simulink model "Pendulum_model_linearization_torque"  (R2016a)
settings: Solver=ode45  StartTime=0.0  StopTime=10  RelTol=1e-3
model workspace: external: MATLAB File C:\Users\Dick\Documents\GitHub\control-system-lab\dick\Matlab\Pendulum simulation\params.m (data not in the file)
values from neighbouring files (symbols this model uses):
  k_m = 50    [linearization_by_hand.m]    (also in params.m = 41.0587; symbolic_derivation.m)
  tau_e = 0.03    [linearization_by_hand.m]    (also in params.m = 0.0312; symbolic_derivation.m)
settings Model: Creator=Nathan  LastModifiedBy=Dick
settings DataIOCC: InitialState=states  LimitDataPoints=on  LoadInitialState=on  SaveFormat=Array
settings DebuggingCC: AllowSymbolicDim=off
settings HardwareCC: ProdBitPerPointer=32  ProdLargestAtomicFloat=None  ProdIntDivRoundTo=Undefined  ProdEndianess=Unspecified  ProdWordSize=32  ProdHWDeviceType=32-bit Generic
settings ModelReferenceCC: PropagateSignalLabelsOutOfModel=off
settings ConfigComp: CovModelRefEnable=Off

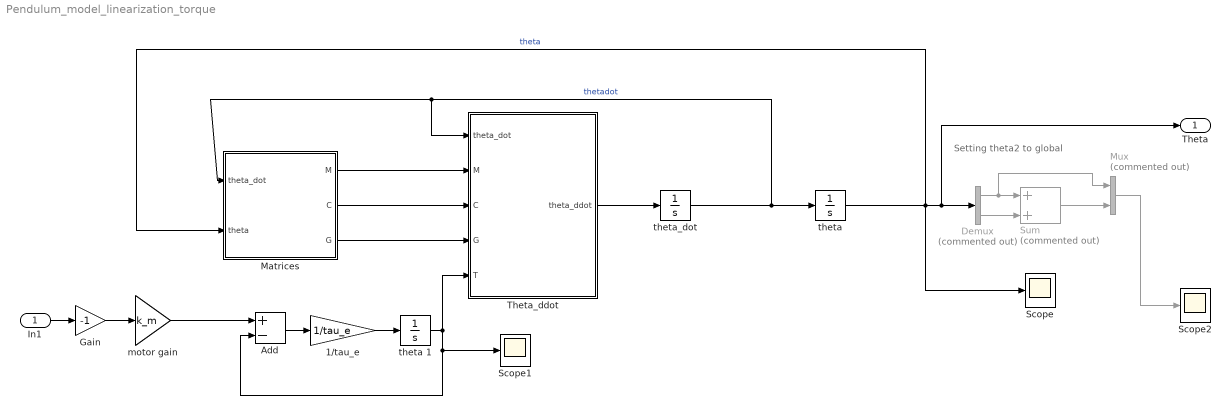
== system Pendulum_model_linearization_torque ==
  note: Setting theta2 to global
  In1 : Inport
  "1/tau_e " : Gain  Gain=1/tau_e
  Add : Sum  Inputs=+-
  Demux : Demux  Commented=on  Outputs=2
  Gain : Gain  Gain=-1
  Matrices : MATLAB Function  TreatAsAtomicUnit=on
  Mux : Mux  Commented=on  Inputs=2
  Scope : Scope
  Scope1 : Scope
  Scope2 : Scope
  Sum : Sum  Commented=on  Inputs=+|+
  "Theta_ddot " : MATLAB Function  TreatAsAtomicUnit=on
  "motor gain " : Gain  Gain=k_m
  "theta " : Integrator
  theta 1 : Integrator  ContinuousStateAttributes='torque'
  "theta_dot " : Integrator
  Theta : Outport
  wires:
  "theta "/1 -> Theta/1, Demux/1, Scope/1, Matrices/2(theta)  "theta"
  "theta_dot "/1 -> "theta "/1, "Theta_ddot "/1(theta_dot), Matrices/1(theta_dot)  "thetadot"
  "Theta_ddot "/1(theta_ddot) -> "theta_dot "/1
  Matrices/3(G) -> "Theta_ddot "/4(G)
  Matrices/2(C) -> "Theta_ddot "/3(C)
  Matrices/1(M) -> "Theta_ddot "/2(M)
  Demux/1 -> Mux/1, Sum/1
  Demux/2 -> Sum/2
  Sum/1 -> Mux/2
  Mux/1 -> Scope2/1
  In1/1 -> Gain/1
  theta 1/1 -> Scope1/1, Add/2, "Theta_ddot "/5(T)
  "1/tau_e "/1 -> theta 1/1
  Add/1 -> "1/tau_e "/1
  "motor gain "/1 -> Add/1
  Gain/1 -> "motor gain "/1

== matlab function Pendulum_model_linearization_torque/Theta_ddot  ==
  data: theta_dot input; M input; C input; G input; theta_ddot output; T input
function theta_ddot = fcn(theta_dot,M,C,G,T)
theta_ddot = [0;0];

theta_ddot = M\[T;0] - M\C*theta_dot - M\G;

== matlab function Pendulum_model_linearization_torque/Matrices ==
  data: theta_dot input; theta input; M output; C output; G output
function [M, C, G] = fcn(theta_dot, theta)

M = zeros(2);
C = zeros(2);
G = [0;0];

% %% Old parameters
% g = 9.81; 
% l1 = 0.1;
% l2 = 0.1;
% m1 = 0.125;
% m2 = 0.05;
% c1 = -0.04; % Keeping it negative results in no motion at all, -0.04 or + 0.04?
% c2 = 0.06;
% I1 = 0.074;
% I2 = 0.00012;
% b1 = 4.8;
% b2 = 0.0002;
% 
% P1 = m1*c1^2+m2*l1^2+I1;
% P2 = m2*c2^2+ I2;
% P3 = m2*l1*c2;
% g1 = (m1*c1+m2*l1)*g;
% g2 = m2*c2*g;

%% New parameters after parameter estimation
g = 9.81; 
l1 = 0.1;
l2 = 0.1;
m1 = 0.125;
m2 = 0.05;
c1 = -0.04; % Keeping it negative results in no motion at all, -0.04 or + 0.04?
c2 = 0.06;
I1 = 0.0029;
I2 = 1e-5*7.8856;
b1 = 5.8039;
b2 = 3.1250e-5;

P1 = m1*c1^2+m2*l1^2+I1;
P2 = m2*c2^2+ I2;
P3 = m2*l1*c2;
g1 = (m1*c1+m2*l1)*g;
g2 = m2*c2*g;


M = [(P1 + P2 + 2*P3*cos(theta(2)))               (P2 + P3*cos(theta(2))) ;
     (P2 + P3*cos(theta(2)))                       P2                   ];
 
 
C = [(b1 - P3*theta_dot(2)*sin(theta(2)))           (-P3*(theta_dot(1)+theta_dot(2))*sin(theta(2))) ;
     (P3*theta_dot(1)*sin(theta(2)))                 b2                                      ];
     
G = [(-g1*sin(theta(1))-g2*sin(theta(1) + theta(2))) ;
      -g2*sin(theta(1)+theta(2))                   ];
